simulink model "TriTiltPro_V3"  (R2019a)
settings: Solver=ode15s  StartTime=0.0  StopTime=1  RelTol=1e-3  EnableMultiTasking=on
undefined symbols (not defined in the file or in its folder): magnitude, sigbuilder_block, X, Y, Z
libraries: sm_lib x405, nesl_utility x28, simulink x13, fl_lib x7, fl_ps_legacy_lib x6, sharedtransform x1, Multibody_Multiphysics_Lib x1
(part 3 of 9)

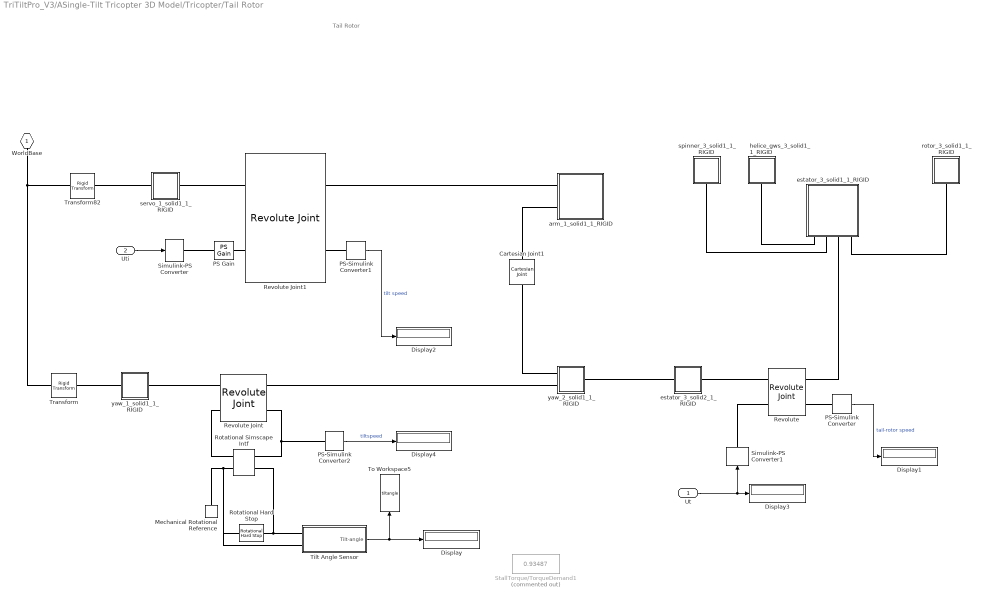
== system TriTiltPro_V3/ASingle-Tilt Tricopter 3D Model/Tricopter/Tail Rotor ==
  note: Tail Rotor
  Ut : Inport
  Uti : Inport  Port=2
  Cartesian Joint1 : sm_lib/Joints/Cartesian Joint  SenseConstraintForce=off  SenseConstraintForceX=off  SenseConstraintForceY=off  SenseConstraintForceZ=off  SenseConstraintTorque=off  SenseConstraintTorqueX=off  SenseConstraintTorqueY=off  SenseConstraintTorqueZ=off  SenseTotalForce=off  SenseTotalForceX=off  SenseTotalForceY=off  SenseTotalForceZ=off  SenseTotalTorque=off  SenseTotalTorqueX=off  SenseTotalTorqueY=off  SenseTotalTorqueZ=off  CompositeWrenchDir=FollowerOnBase  CompositeWrenchFrame=BaseFrame  PxEquilibriumPosition=0  PxEquilibriumPositionUnits=m  PxSpringStiffness=0  PxSpringStiffnessUnits=N/m  PxDampingCoefficient=0  PxDampingCoefficientUnits=N/(m/s)  PxTorqueActuationMode=NoTorque  PxMotionActuationMode=ComputedMotion  PxSensePosition=off  PxSenseVelocity=off  PxSenseAcceleration=off  PxSenseTorqueForce=off  PxSenseLowerLimitTorqueForce=off  PxSenseUpperLimitTorqueForce=off  PxLowerLimitSpecify=off  PxLowerLimitBound=-1  PxLowerLimitBoundUnits=m  PxLowerLimitStiffness=1e6  PxLowerLimitStiffnessUnits=N/m  PxLowerLimitDamping=1e3  PxLowerLimitDampingUnits=N/(m/s)  PxLowerLimitTransitionRegionWidth=1e-4  PxLowerLimitTransitionRegionWidthUnits=m  PxUpperLimitSpecify=off  PxUpperLimitBound=1  PxUpperLimitBoundUnits=m  PxUpperLimitStiffness=1e6  PxUpperLimitStiffnessUnits=N/m  PxUpperLimitDamping=1e3  PxUpperLimitDampingUnits=N/(m/s)  PxUpperLimitTransitionRegionWidth=1e-4  PxUpperLimitTransitionRegionWidthUnits=m  PxPositionTargetSpecify=off  PxPositionTargetPriority=Low  PxPositionTargetValue=-0.0011181976595044071  PxPositionTargetValueUnits=m  PxVelocityTargetSpecify=off  PxVelocityTargetPriority=High  PxVelocityTargetValue=0  PxVelocityTargetValueUnits=m/s  PyEquilibriumPosition=0  PyEquilibriumPositionUnits=m  PySpringStiffness=0  PySpringStiffnessUnits=N/m  PyDampingCoefficient=0  PyDampingCoefficientUnits=N/(m/s)  PyTorqueActuationMode=NoTorque  PyMotionActuationMode=ComputedMotion  PySensePosition=off  PySenseVelocity=off  PySenseAcceleration=off  PySenseTorqueForce=off  PySenseLowerLimitTorqueForce=off  PySenseUpperLimitTorqueForce=off  PyLowerLimitSpecify=off  PyLowerLimitBound=-1  PyLowerLimitBoundUnits=m  PyLowerLimitStiffness=1e6  PyLowerLimitStiffnessUnits=N/m  PyLowerLimitDamping=1e3  PyLowerLimitDampingUnits=N/(m/s)  PyLowerLimitTransitionRegionWidth=1e-4  PyLowerLimitTransitionRegionWidthUnits=m  PyUpperLimitSpecify=off  PyUpperLimitBound=1  PyUpperLimitBoundUnits=m  PyUpperLimitStiffness=1e6  PyUpperLimitStiffnessUnits=N/m  PyUpperLimitDamping=1e3  PyUpperLimitDampingUnits=N/(m/s)  PyUpperLimitTransitionRegionWidth=1e-4  PyUpperLimitTransitionRegionWidthUnits=m  PyPositionTargetSpecify=off  PyPositionTargetPriority=Low  PyPositionTargetValue=7.2724548069575946e-05  PyPositionTargetValueUnits=m  PyVelocityTargetSpecify=off  PyVelocityTargetPriority=High  PyVelocityTargetValue=0  PyVelocityTargetValueUnits=m/s  PzEquilibriumPosition=0  PzEquilibriumPositionUnits=m  PzSpringStiffness=0  PzSpringStiffnessUnits=N/m  PzDampingCoefficient=0  PzDampingCoefficientUnits=N/(m/s)  PzTorqueActuationMode=NoTorque  PzMotionActuationMode=ComputedMotion  PzSensePosition=off  PzSenseVelocity=off  PzSenseAcceleration=off  PzSenseTorqueForce=off  PzSenseLowerLimitTorqueForce=off  PzSenseUpperLimitTorqueForce=off  PzLowerLimitSpecify=off  PzLowerLimitBound=-1  PzLowerLimitBoundUnits=m  PzLowerLimitStiffness=1e6  PzLowerLimitStiffnessUnits=N/m  PzLowerLimitDamping=1e3  PzLowerLimitDampingUnits=N/(m/s)  PzLowerLimitTransitionRegionWidth=1e-4  PzLowerLimitTransitionRegionWidthUnits=m  PzUpperLimitSpecify=off  PzUpperLimitBound=1  PzUpperLimitBoundUnits=m  PzUpperLimitStiffness=1e6  PzUpperLimitStiffnessUnits=N/m  PzUpperLimitDamping=1e3  PzUpperLimitDampingUnits=N/(m/s)  PzUpperLimitTransitionRegionWidth=1e-4  PzUpperLimitTransitionRegionWidthUnits=m  PzPositionTargetSpecify=on  PzPositionTargetPriority=High  PzPositionTargetValue=-3.6271878084718665e-16  PzPositionTargetValueUnits=m  PzVelocityTargetSpecify=off  PzVelocityTargetPriority=High  PzVelocityTargetValue=0  PzVelocityTargetValueUnits=m/s
  Display{,1..4} (5 alike) : Display
  Mechanical Rotational Reference : fl_lib/Mechanical/Rotational Elements/Mechanical Rotational Reference
  PS Gain : fl_lib/Physical Signals/Functions/PS Gain  gain=1
  PS-Simulink Converter : nesl_utility/PS-Simulink Converter  PhysicalDomain=network_engine_domain  SubClassName=ps_output  LeftPortType=input  RightPortType=output  PseudoPeriodic=off  Frequencies=[]  Unit=rpm  AffineConversion=off
  PS-Simulink Converter1 : nesl_utility/PS-Simulink Converter  PhysicalDomain=network_engine_domain  SubClassName=ps_output  LeftPortType=input  RightPortType=output  PseudoPeriodic=off  Frequencies=[]  Unit=rpm  AffineConversion=off
  PS-Simulink Converter2 : nesl_utility/PS-Simulink Converter  PhysicalDomain=network_engine_domain  SubClassName=ps_output  LeftPortType=input  RightPortType=output  PseudoPeriodic=off  Frequencies=[]  Unit=rpm  AffineConversion=off
  Revolute : sm_lib/Joints/Revolute Joint  SenseConstraintForce=off  SenseConstraintForceX=off  SenseConstraintForceY=off  SenseConstraintForceZ=off  SenseConstraintTorque=off  SenseConstraintTorqueX=off  SenseConstraintTorqueY=off  SenseConstraintTorqueZ=off  SenseTotalForce=off  SenseTotalForceX=off  SenseTotalForceY=off  SenseTotalForceZ=off  SenseTotalTorque=off  SenseTotalTorqueX=off  SenseTotalTorqueY=off  SenseTotalTorqueZ=off  CompositeWrenchDir=FollowerOnBase  CompositeWrenchFrame=BaseFrame  EquilibriumPosition=0  EquilibriumPositionUnits=rad  SpringStiffness=0  SpringStiffnessUnits=m*N/rad  DampingCoefficient=0  DampingCoefficientUnits=m*s*N/rad  TorqueActuationMode=InputTorque  MotionActuationMode=ComputedMotion  SensePosition=off  SenseVelocity=on  SenseAcceleration=off  SenseTorqueForce=off  SenseLowerLimitTorqueForce=off  SenseUpperLimitTorqueForce=off  LowerLimitSpecify=off  LowerLimitBound=-90  LowerLimitBoundUnits=deg  LowerLimitStiffness=1e4  LowerLimitStiffnessUnits=N*m/deg  LowerLimitDamping=10  LowerLimitDampingUnits=N*m/(deg/s)  LowerLimitTransitionRegionWidth=0.1  LowerLimitTransitionRegionWidthUnits=deg  UpperLimitSpecify=off  UpperLimitBound=90  UpperLimitBoundUnits=deg  UpperLimitStiffness=1e4  UpperLimitStiffnessUnits=N*m/deg  UpperLimitDamping=10  UpperLimitDampingUnits=N*m/(deg/s)  UpperLimitTransitionRegionWidth=0.1  UpperLimitTransitionRegionWidthUnits=deg  PositionTargetSpecify=on  PositionTargetPriority=Low  PositionTargetValue=57.946376852281944  PositionTargetValueUnits=deg  VelocityTargetSpecify=off  VelocityTargetPriority=High  VelocityTargetValue=0  VelocityTargetValueUnits=deg/s
  Revolute Joint : sm_lib/Joints/Revolute Joint  SenseConstraintForce=off  SenseConstraintForceX=off  SenseConstraintForceY=off  SenseConstraintForceZ=off  SenseConstraintTorque=off  SenseConstraintTorqueX=off  SenseConstraintTorqueY=off  SenseConstraintTorqueZ=off  SenseTotalForce=off  SenseTotalForceX=off  SenseTotalForceY=off  SenseTotalForceZ=off  SenseTotalTorque=off  SenseTotalTorqueX=off  SenseTotalTorqueY=off  SenseTotalTorqueZ=off  CompositeWrenchDir=FollowerOnBase  CompositeWrenchFrame=BaseFrame  EquilibriumPosition=0  EquilibriumPositionUnits=deg  SpringStiffness=0  SpringStiffnessUnits=N*m/deg  DampingCoefficient=0  DampingCoefficientUnits=N*m/(deg/s)  TorqueActuationMode=InputTorque  MotionActuationMode=ComputedMotion  SensePosition=off  SenseVelocity=on  SenseAcceleration=off  SenseTorqueForce=off  SenseLowerLimitTorqueForce=off  SenseUpperLimitTorqueForce=off  LowerLimitSpecify=off  LowerLimitBound=-90  LowerLimitBoundUnits=deg  LowerLimitStiffness=1e4  LowerLimitStiffnessUnits=N*m/deg  LowerLimitDamping=10  LowerLimitDampingUnits=N*m/(deg/s)  LowerLimitTransitionRegionWidth=0.1  LowerLimitTransitionRegionWidthUnits=deg  UpperLimitSpecify=off  UpperLimitBound=90  UpperLimitBoundUnits=deg  UpperLimitStiffness=1e4  UpperLimitStiffnessUnits=N*m/deg  UpperLimitDamping=10  UpperLimitDampingUnits=N*m/(deg/s)  UpperLimitTransitionRegionWidth=0.1  UpperLimitTransitionRegionWidthUnits=deg  PositionTargetSpecify=off  PositionTargetPriority=Low  PositionTargetValue=0  PositionTargetValueUnits=deg  VelocityTargetSpecify=off  VelocityTargetPriority=High  VelocityTargetValue=0  VelocityTargetValueUnits=deg/s
  Revolute Joint1 : sm_lib/Joints/Revolute Joint  SenseConstraintForce=off  SenseConstraintForceX=off  SenseConstraintForceY=off  SenseConstraintForceZ=off  SenseConstraintTorque=off  SenseConstraintTorqueX=off  SenseConstraintTorqueY=off  SenseConstraintTorqueZ=off  SenseTotalForce=off  SenseTotalForceX=off  SenseTotalForceY=off  SenseTotalForceZ=off  SenseTotalTorque=off  SenseTotalTorqueX=off  SenseTotalTorqueY=off  SenseTotalTorqueZ=off  CompositeWrenchDir=FollowerOnBase  CompositeWrenchFrame=BaseFrame  EquilibriumPosition=0  EquilibriumPositionUnits=deg  SpringStiffness=0  SpringStiffnessUnits=N*m/deg  DampingCoefficient=0  DampingCoefficientUnits=N*m/(deg/s)  TorqueActuationMode=InputTorque  MotionActuationMode=ComputedMotion  SensePosition=off  SenseVelocity=on  SenseAcceleration=off  SenseTorqueForce=off  SenseLowerLimitTorqueForce=off  SenseUpperLimitTorqueForce=off  LowerLimitSpecify=off  LowerLimitBound=-90  LowerLimitBoundUnits=deg  LowerLimitStiffness=1e4  LowerLimitStiffnessUnits=N*m/deg  LowerLimitDamping=10  LowerLimitDampingUnits=N*m/(deg/s)  LowerLimitTransitionRegionWidth=0.1  LowerLimitTransitionRegionWidthUnits=deg  UpperLimitSpecify=off  UpperLimitBound=90  UpperLimitBoundUnits=deg  UpperLimitStiffness=1e4  UpperLimitStiffnessUnits=N*m/deg  UpperLimitDamping=10  UpperLimitDampingUnits=N*m/(deg/s)  UpperLimitTransitionRegionWidth=0.1  UpperLimitTransitionRegionWidthUnits=deg  PositionTargetSpecify=on  PositionTargetPriority=Low  PositionTargetValue=7.4422433437709268  PositionTargetValueUnits=deg  VelocityTargetSpecify=off  VelocityTargetPriority=High  VelocityTargetValue=0  VelocityTargetValueUnits=deg/s
  Rotational Simscape Intf : Multibody_Multiphysics_Lib/Interfaces/Rotational Simscape Intf  SystemSampleTime=-1
      settings: SourceProductName=Simscape Multibody Multiphysics Library
  Rotational Hard Stop : fl_lib/Mechanical/Rotational Elements/Rotational Hard Stop  upper_bnd=225 deg  lower_bnd=135 deg  stiff_up=2e6 N*m/rad  stiff_low=2e6 N*m/rad  D_up=0.000001 N*m/(rad/s)  D_low=0.000001 N*m/(rad/s)  model=3  transition=0.001 rad  w_specify=off  w_priority=High  w=0 rad/s  w_nominal_specify=off  w_nominal_unit=rad/s  w_nominal_value=1  t_specify=off  t_priority=High  t=0 N*m  t_nominal_specify=off  t_nominal_unit=N*m  t_nominal_value=1  phi_specify=on  phi_priority=High  phi=180 deg  phi_nominal_specify=off  phi_nominal_unit=rad  phi_nominal_value=1
      settings: SourceProductName=Simscape  SourceProductBaseCode=SS
  Simulink-PS Converter : nesl_utility/Simulink-PS Converter  PhysicalDomain=network_engine_domain  SubClassName=ps_input  LeftPortType=input  RightPortType=output  PseudoPeriodic=off  Frequencies=[]  NoiseDistribution=none  NoiseParameters=[]  Unit=N*m  AffineConversion=off  FilteringAndDerivatives=zero  SimscapeFilterOrder=1  InputFilterTimeConstant=0.001  UdotUserProvided=1
  Simulink-PS Converter1 : nesl_utility/Simulink-PS Converter  PhysicalDomain=network_engine_domain  SubClassName=ps_input  LeftPortType=input  RightPortType=output  PseudoPeriodic=off  Frequencies=[]  NoiseDistribution=none  NoiseParameters=[]  Unit=N*m  AffineConversion=off  FilteringAndDerivatives=zero  SimscapeFilterOrder=1  InputFilterTimeConstant=0.001  UdotUserProvided=1
  StallTorque/TorqueDemand1 : Constant  Commented=on  Value=0.93487
  Tilt Angle Sensor : Subsystem
  To Workspace5 : ToWorkspace  VariableName=tiltangle  SampleTime=-1
  Transform : sm_lib/Frames and Transforms/Rigid Transform  TranslationMethod=None  TranslationStandardOffset=0  TranslationLengthUnit=m  TranslationStandardAxis=+Z  TranslationCartesianOffset=[0 0 0]  TranslationROffset=0  TranslationROffsetUnits=m  TranslationZOffset=0  TranslationZOffsetUnits=m  TranslationThetaOffset=0  TranslationThetaOffsetUnits=deg  RotationMethod=None  RotationAngleUnits=deg  RotationStandardAxis=+Z  RotationAngle=0.0  RotationArbitraryAxis=[0 0 1]  FollAlignAxisA=+X  BaseAlignAxisA=+Y  FollAlignAxisB=+Y  BaseAlignAxisB=+Z  RotationSequenceAxes=FollowerAxes  RotationSequence=XYX  RotationSequenceAngles=[0 0 0]  RotationSequenceAnglesUnits=deg  RotationMatrix=[1 0 0; 0 1 0; 0 0 1]
  Transform82 : sm_lib/Frames and Transforms/Rigid Transform  TranslationMethod=None  TranslationStandardOffset=0  TranslationLengthUnit=m  TranslationStandardAxis=+Z  TranslationCartesianOffset=[0 0 0]  TranslationROffset=0  TranslationROffsetUnits=m  TranslationZOffset=0  TranslationZOffsetUnits=m  TranslationThetaOffset=0  TranslationThetaOffsetUnits=deg  RotationMethod=None  RotationAngleUnits=deg  RotationStandardAxis=+Z  RotationAngle=0.0  RotationArbitraryAxis=[0 0 1]  FollAlignAxisA=+X  BaseAlignAxisA=+Y  FollAlignAxisB=+Y  BaseAlignAxisB=+Z  RotationSequenceAxes=FollowerAxes  RotationSequence=XYX  RotationSequenceAngles=[0 0 0]  RotationSequenceAnglesUnits=deg  RotationMatrix=[1 0 0; 0 1 0; 0 0 1]
  arm_1_solid1_1_RIGID : Subsystem
  estator_3_solid1_1_RIGID : Subsystem
  estator_3_solid2_1_RIGID : Subsystem
  helice_gws_3_solid1_1_RIGID : Subsystem
  rotor_3_solid1_1_RIGID : Subsystem
  servo_1_solid1_1_RIGID : Subsystem
  spinner_3_solid1_1_RIGID : Subsystem
  yaw_1_solid1_1_RIGID : Subsystem
  yaw_2_solid1_1_RIGID : Subsystem
  WorldBase : PMIOPort  Side=Right
  wires:
  Tilt Angle Sensor/1(Tilt-angle) -> To Workspace5/1, Display/1
  PS-Simulink Converter/1 -> Display1/1  "tail-rotor speed"
  Uti/1 -> Simulink-PS Converter/1
  Ut/1 -> Display3/1, Simulink-PS Converter1/1
  PS-Simulink Converter1/1 -> Display2/1  "tilt speed"
  PS-Simulink Converter2/1 -> Display4/1  "tiltspeed"
  connections:
  Transform/RConn1 -- yaw_1_solid1_1_RIGID/LConn1
  estator_3_solid2_1_RIGID/LConn1 -- yaw_2_solid1_1_RIGID/RConn1
  Transform82/RConn1 -- servo_1_solid1_1_RIGID/LConn1
  WorldBase/RConn1 -- Transform82/LConn1 -- Transform/LConn1
  Revolute Joint/LConn1 -- yaw_1_solid1_1_RIGID/RConn1
  Revolute Joint/RConn1 -- yaw_2_solid1_1_RIGID/LConn2
  Revolute Joint1/LConn1 -- servo_1_solid1_1_RIGID/RConn1
  Revolute Joint1/RConn1 -- arm_1_solid1_1_RIGID/LConn1
  Tilt Angle Sensor/LConn2 -- Rotational Hard Stop/RConn1 -- Rotational Simscape Intf/LConn2 -- Mechanical Rotational Reference/LConn1
  estator_3_solid2_1_RIGID/RConn1 -- Revolute/LConn1
  PS-Simulink Converter/LConn1 -- Revolute/RConn2
  PS Gain/RConn1 -- Revolute Joint1/LConn2
  Simulink-PS Converter/RConn1 -- PS Gain/LConn1
  arm_1_solid1_1_RIGID/LConn2 -- Cartesian Joint1/LConn1
  Tilt Angle Sensor/LConn1 -- Rotational Simscape Intf/RConn2 -- Rotational Hard Stop/LConn1
  Revolute Joint/RConn2 -- Rotational Simscape Intf/RConn1 -- PS-Simulink Converter2/LConn1
  Rotational Simscape Intf/LConn1 -- Revolute Joint/LConn2
  Simulink-PS Converter1/RConn1 -- Revolute/LConn2
  PS-Simulink Converter1/LConn1 -- Revolute Joint1/RConn2
  Cartesian Joint1/RConn1 -- yaw_2_solid1_1_RIGID/LConn1
  helice_gws_3_solid1_1_RIGID/LConn1 -- estator_3_solid1_1_RIGID/LConn1
  spinner_3_solid1_1_RIGID/LConn1 -- estator_3_solid1_1_RIGID/LConn2
  rotor_3_solid1_1_RIGID/LConn1 -- estator_3_solid1_1_RIGID/LConn4
  estator_3_solid1_1_RIGID/LConn3 -- Revolute/RConn1

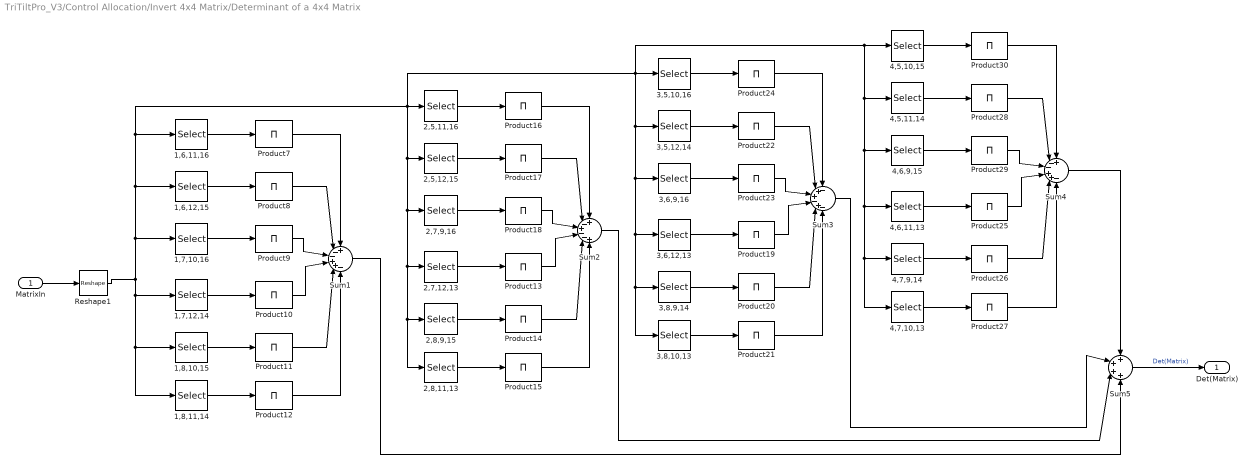
== system TriTiltPro_V3/Control Allocation/Invert 4x4 Matrix/Determinant of a 4x4 Matrix ==
  MatrixIn : Inport
  1,6,11,16 : Selector  InputPortWidth=16  IndexOptions=Index vector (dialog)  Indices=[1 6 11 16]  OutputSizes=1
  1,6,12,15 : Selector  InputPortWidth=16  IndexOptions=Index vector (dialog)  Indices=[1 6 12 15]  OutputSizes=1
  1,7,10,16 : Selector  InputPortWidth=16  IndexOptions=Index vector (dialog)  Indices=[1 7 10 16]  OutputSizes=1
  1,7,12,14 : Selector  InputPortWidth=16  IndexOptions=Index vector (dialog)  Indices=[1 7 10 16]  OutputSizes=1
  1,8,10,15 : Selector  InputPortWidth=16  IndexOptions=Index vector (dialog)  Indices=[1 7 10 16]  OutputSizes=1
  1,8,11,14 : Selector  InputPortWidth=16  IndexOptions=Index vector (dialog)  Indices=[1 7 10 16]  OutputSizes=1
  2,5,11,16 : Selector  InputPortWidth=16  IndexOptions=Index vector (dialog)  Indices=[2 5 11 16]  OutputSizes=1
  2,5,12,15 : Selector  InputPortWidth=16  IndexOptions=Index vector (dialog)  Indices=[2 5 12 15]  OutputSizes=1
  2,7,12,13 : Selector  InputPortWidth=16  IndexOptions=Index vector (dialog)  Indices=[2 7 12 13]  OutputSizes=1
  2,7,9,16 : Selector  InputPortWidth=16  IndexOptions=Index vector (dialog)  Indices=[2 7 9 16]  OutputSizes=1
  2,8,11,13 : Selector  InputPortWidth=16  IndexOptions=Index vector (dialog)  Indices=[2 8 11 13]  OutputSizes=1
  2,8,9,15 : Selector  InputPortWidth=16  IndexOptions=Index vector (dialog)  Indices=[2 8 9 15]  OutputSizes=1
  3,5,10,16 : Selector  InputPortWidth=16  IndexOptions=Index vector (dialog)  Indices=[3 5 10 16]  OutputSizes=1
  3,5,12,14 : Selector  InputPortWidth=16  IndexOptions=Index vector (dialog)  Indices=[3 5 12 14]  OutputSizes=1
  3,6,12,13 : Selector  InputPortWidth=16  IndexOptions=Index vector (dialog)  Indices=[3 6 12 13]  OutputSizes=1
  3,6,9,16 : Selector  InputPortWidth=16  IndexOptions=Index vector (dialog)  Indices=[3 6 9 16]  OutputSizes=1
  3,8,10,13 : Selector  InputPortWidth=16  IndexOptions=Index vector (dialog)  Indices=[3 8 10 13]  OutputSizes=1
  3,8,9,14 : Selector  InputPortWidth=16  IndexOptions=Index vector (dialog)  Indices=[3 8 9 14]  OutputSizes=1
  4,5,10,15 : Selector  InputPortWidth=16  IndexOptions=Index vector (dialog)  Indices=[4 5 10 15]  OutputSizes=1
  4,5,11,14 : Selector  InputPortWidth=16  IndexOptions=Index vector (dialog)  Indices=[4 5 11 14]  OutputSizes=1
  4,6,11,13 : Selector  InputPortWidth=16  IndexOptions=Index vector (dialog)  Indices=[4 6 11 13]  OutputSizes=1
  4,6,9,15 : Selector  InputPortWidth=16  IndexOptions=Index vector (dialog)  Indices=[4 6 9 15]  OutputSizes=1
  4,7,10,13 : Selector  InputPortWidth=16  IndexOptions=Index vector (dialog)  Indices=[4 7 10 13]  OutputSizes=1
  4,7,9,14 : Selector  InputPortWidth=16  IndexOptions=Index vector (dialog)  Indices=[4 7 9 14]  OutputSizes=1
  Product{7..30} (24 alike) : Product  Inputs=1  SaturateOnIntegerOverflow=on  OutDataTypeStr=Inherit: Same as first input
  Reshape1 : Reshape  OutputDimensionality=Row vector (2-D)  OutputDimensions=[4,4]
  Sum1 : Sum  Inputs=+--++-  SaturateOnIntegerOverflow=on
  Sum2 : Sum  Inputs=+-+--+  SaturateOnIntegerOverflow=on
  Sum3 : Sum  Inputs=-++-+-  SaturateOnIntegerOverflow=on
  Sum4 : Sum  Inputs=+--++-  SaturateOnIntegerOverflow=on
  Sum5 : Sum  Inputs=++++  SaturateOnIntegerOverflow=on
  Det(Matrix) : Outport
  wires:
  Product8/1 -> Sum1/2
  1,6,11,16/1 -> Product7/1
  3,5,10,16/1 -> Product24/1
  Reshape1/1 -> 1,6,12,15/1, 3,5,12,14/1, 3,8,10,13/1, 3,8,9,14/1, 3,6,12,13/1, 3,6,9,16/1, 4,6,9,15/1, 4,7,10,13/1, 4,7,9,14/1, 4,6,11,13/1, 4,5,11,14/1, 4,5,10,15/1, 3,5,10,16/1, 2,7,9,16/1, 2,8,11,13/1, 2,8,9,15/1, 2,7,12,13/1, 2,5,12,15/1, 2,5,11,16/1, 1,6,11,16/1, 1,7,10,16/1, 1,7,12,14/1, 1,8,11,14/1, 1,8,10,15/1
  1,8,10,15/1 -> Product11/1
  Product10/1 -> Sum1/4
  1,7,10,16/1 -> Product9/1
  Product28/1 -> Sum4/2
  Product25/1 -> Sum4/4
  4,7,10,13/1 -> Product27/1
  Product26/1 -> Sum4/5
  4,6,11,13/1 -> Product25/1
  Product29/1 -> Sum4/3
  4,7,9,14/1 -> Product26/1
  4,6,9,15/1 -> Product29/1
  Product30/1 -> Sum4/1
  4,5,10,15/1 -> Product30/1
  4,5,11,14/1 -> Product28/1
  Product27/1 -> Sum4/6
  2,8,9,15/1 -> Product14/1
  Product13/1 -> Sum2/4
  Product14/1 -> Sum2/5
  1,7,12,14/1 -> Product10/1
  Product17/1 -> Sum2/2
  2,7,12,13/1 -> Product13/1
  Product18/1 -> Sum2/3
  Product15/1 -> Sum2/6
  2,7,9,16/1 -> Product18/1
  2,5,11,16/1 -> Product16/1
  Product16/1 -> Sum2/1
  2,5,12,15/1 -> Product17/1
  2,8,11,13/1 -> Product15/1
  Sum4/1 -> Sum5/1
  1,6,12,15/1 -> Product8/1
  Product11/1 -> Sum1/5
  Sum5/1 -> Det(Matrix)/1  "Det(Matrix)"
  Sum3/1 -> Sum5/2
  Sum2/1 -> Sum5/3
  Product24/1 -> Sum3/1
  Sum1/1 -> Sum5/4
  Product9/1 -> Sum1/3
  Product7/1 -> Sum1/1
  Product23/1 -> Sum3/3
  3,8,9,14/1 -> Product20/1
  Product22/1 -> Sum3/2
  Product19/1 -> Sum3/4
  3,8,10,13/1 -> Product21/1
  Product20/1 -> Sum3/5
  Product21/1 -> Sum3/6
  3,6,12,13/1 -> Product19/1
  3,5,12,14/1 -> Product22/1
  3,6,9,16/1 -> Product23/1
  1,8,11,14/1 -> Product12/1
  Product12/1 -> Sum1/6
  MatrixIn/1 -> Reshape1/1

== system TriTiltPro_V3/Reference Inputs/Inputs1/Signal Builder ==
  Demux : Demux  Tag=STV Demux
  FromWs : FromWorkspace  Tag=STV FromWs  VariableName=tuvar  SampleTime=0
      SigBuilderData=|
      | common.afterFinalStr = 'Extrapolate'
      | common.sampleTime = '0'
      | dataSet.timeRange = [0 2]
      | dataSet.name = 'Group 1'
      | sbobj.Groups.Name = 'Group 1'
      | sbobj.Groups.Signals(1).Name = 'Test Altitude'
      | sbobj.Groups.Signals(1).XData = [0 0.2 0.4 0.6 0.8 2]
      | sbobj.Groups.Signals(1).YData = [0 0 0 0 0 0]
      | sbobj.Groups.Signals(2).Name = 'Test Roll'
      | sbobj.Groups.Signals(2).XData = [0 0.995 2]
      | sbobj.Groups.Signals(2).YData = [0 0 0]
      | sbobj.Groups.Signals(3).Name = 'Test Pitch'
      | sbobj.Groups.Signals(3).XData = [0 2]
      | sbobj.Groups.Signals(3).YData = [0 0]
      | sbobj.Groups.Signals(4).Name = 'Test Yaw'
      | sbobj.Groups.Signals(4).XData = [0 2]
      | sbobj.Groups.Signals(4).YData = [0 0]
      | sbobj.Groups.TimeRange = [0 2]
  Test Altitude : Outport  Tag=STV Outport
  Test Roll : Outport  Tag=STV Outport  Port=2
  Test Pitch : Outport  Tag=STV Outport  Port=3
  Test Yaw : Outport  Tag=STV Outport  Port=4
  wires:
  FromWs/1 -> Demux/1
  Demux/1 -> Test Altitude/1
  Demux/2 -> Test Roll/1
  Demux/3 -> Test Pitch/1
  Demux/4 -> Test Yaw/1

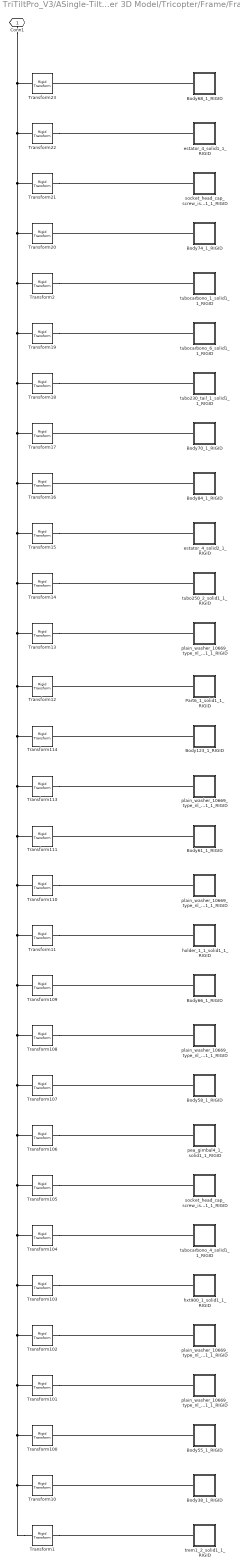
== system TriTiltPro_V3/ASingle-Tilt Tricopter 3D Model/Tricopter/Frame/Frame B ==
  Body123_1_RIGID : Subsystem
  Body38_1_RIGID : Subsystem
  Body55_1_RIGID : Subsystem
  Body58_1_RIGID : Subsystem
  Body61_1_RIGID : Subsystem
  Body66_1_RIGID : Subsystem
  Body68_1_RIGID : Subsystem
  Body70_1_RIGID : Subsystem
  Body74_1_RIGID : Subsystem
  Body84_1_RIGID : Subsystem
  Part6_1_solid1_1_RIGID : Subsystem
  Transform{1..2,10..23,100..111,113..114} (30 alike) : sm_lib/Frames and Transforms/Rigid Transform  TranslationMethod=None  TranslationStandardOffset=0  TranslationLengthUnit=m  TranslationStandardAxis=+Z  TranslationCartesianOffset=[0 0 0]  TranslationROffset=0  TranslationROffsetUnits=m  TranslationZOffset=0  TranslationZOffsetUnits=m  TranslationThetaOffset=0  TranslationThetaOffsetUnits=deg  RotationMethod=None  RotationAngleUnits=deg  RotationStandardAxis=+Z  RotationAngle=0.0  RotationArbitraryAxis=[0 0 1]  FollAlignAxisA=+X  BaseAlignAxisA=+Y  FollAlignAxisB=+Y  BaseAlignAxisB=+Z  RotationSequenceAxes=FollowerAxes  RotationSequence=XYX  RotationSequenceAngles=[0 0 0]  RotationSequenceAnglesUnits=deg  RotationMatrix=[1 0 0; 0 1 0; 0 0 1]
  estator_4_solid1_1_RIGID : Subsystem
  estator_4_solid2_1_RIGID : Subsystem
  holder_1_1_solid1_1_RIGID : Subsystem
  hxt900_1_solid1_1_RIGID : Subsystem
  pea_gimbal4_1_solid1_1_RIGID : Subsystem
  plain_washer_10669_type_nl_iso_10_solid1_1_RIGID : Subsystem
  plain_washer_10669_type_nl_iso_11_solid1_1_RIGID : Subsystem
  plain_washer_10669_type_nl_iso_12_solid1_1_RIGID : Subsystem
  plain_washer_10669_type_nl_iso_13_solid1_1_RIGID : Subsystem
  plain_washer_10669_type_nl_iso_14_solid1_1_RIGID : Subsystem
  plain_washer_10669_type_nl_iso_4_solid1_1_RIGID : Subsystem
  socket_head_cap_screw_iso_3_solid1_1_RIGID : Subsystem
  socket_head_cap_screw_iso_4_solid1_1_RIGID : Subsystem
  trem1_2_solid1_1_RIGID : Subsystem
  tubo230_tail_1_solid1_1_RIGID : Subsystem
  tubo250_2_solid1_1_RIGID : Subsystem
  tubocarbono_1_solid1_1_RIGID : Subsystem
  tubocarbono_4_solid1_1_RIGID : Subsystem
  tubocarbono_6_solid1_1_RIGID : Subsystem
  Conn1 : PMIOPort  Side=Right
  connections:
  Transform19/RConn1 -- tubocarbono_6_solid1_1_RIGID/LConn1
  Transform21/RConn1 -- socket_head_cap_screw_iso_3_solid1_1_RIGID/LConn1
  Body74_1_RIGID/LConn1 -- Transform20/RConn1
  Transform22/RConn1 -- estator_4_solid1_1_RIGID/LConn1
  Body68_1_RIGID/LConn1 -- Transform23/RConn1
  Part6_1_solid1_1_RIGID/LConn1 -- Transform12/RConn1
  Transform13/RConn1 -- plain_washer_10669_type_nl_iso_10_solid1_1_RIGID/LConn1
  Transform14/RConn1 -- tubo250_2_solid1_1_RIGID/LConn1
  Transform11/RConn1 -- holder_1_1_solid1_1_RIGID/LConn1
  Transform15/RConn1 -- estator_4_solid2_1_RIGID/LConn1
  Body84_1_RIGID/LConn1 -- Transform16/RConn1
  Body38_1_RIGID/LConn1 -- Transform10/RConn1
  Body70_1_RIGID/LConn1 -- Transform17/RConn1
  Transform18/RConn1 -- tubo230_tail_1_solid1_1_RIGID/LConn1
  Transform1/RConn1 -- trem1_2_solid1_1_RIGID/LConn1
  Transform2/RConn1 -- tubocarbono_1_solid1_1_RIGID/LConn1
  Transform103/RConn1 -- hxt900_1_solid1_1_RIGID/LConn1
  Transform110/RConn1 -- plain_washer_10669_type_nl_iso_11_solid1_1_RIGID/LConn1
  Body58_1_RIGID/LConn1 -- Transform107/RConn1
  Transform105/RConn1 -- socket_head_cap_screw_iso_4_solid1_1_RIGID/LConn1
  Transform113/RConn1 -- plain_washer_10669_type_nl_iso_4_solid1_1_RIGID/LConn1
  Body123_1_RIGID/LConn1 -- Transform114/RConn1
  Transform102/RConn1 -- plain_washer_10669_type_nl_iso_13_solid1_1_RIGID/LConn1
  Body55_1_RIGID/LConn1 -- Transform100/RConn1
  Transform101/RConn1 -- plain_washer_10669_type_nl_iso_14_solid1_1_RIGID/LConn1
  Body66_1_RIGID/LConn1 -- Transform109/RConn1
  Transform106/RConn1 -- pea_gimbal4_1_solid1_1_RIGID/LConn1
  Body61_1_RIGID/LConn1 -- Transform111/RConn1
  Transform104/RConn1 -- tubocarbono_4_solid1_1_RIGID/LConn1
  Transform108/RConn1 -- plain_washer_10669_type_nl_iso_12_solid1_1_RIGID/LConn1
  Transform1/LConn1 -- Transform10/LConn1 -- Transform100/LConn1 -- Transform101/LConn1 -- Transform102/LConn1 -- Transform103/LConn1 -- Transform104/LConn1 -- Transform105/LConn1 -- Transform106/LConn1 -- Transform107/LConn1 -- Transform108/LConn1 -- Transform109/LConn1 -- Transform11/LConn1 -- Transform110/LConn1 -- Transform111/LConn1 -- Transform113/LConn1 -- Transform114/LConn1 -- Transform12/LConn1 -- Transform13/LConn1 -- Transform14/LConn1 -- Transform15/LConn1 -- Transform16/LConn1 -- Transform17/LConn1 -- Transform18/LConn1 -- Transform19/LConn1 -- Transform2/LConn1 -- Transform20/LConn1 -- Transform21/LConn1 -- Transform22/LConn1 -- Transform23/LConn1 -- Conn1/RConn1

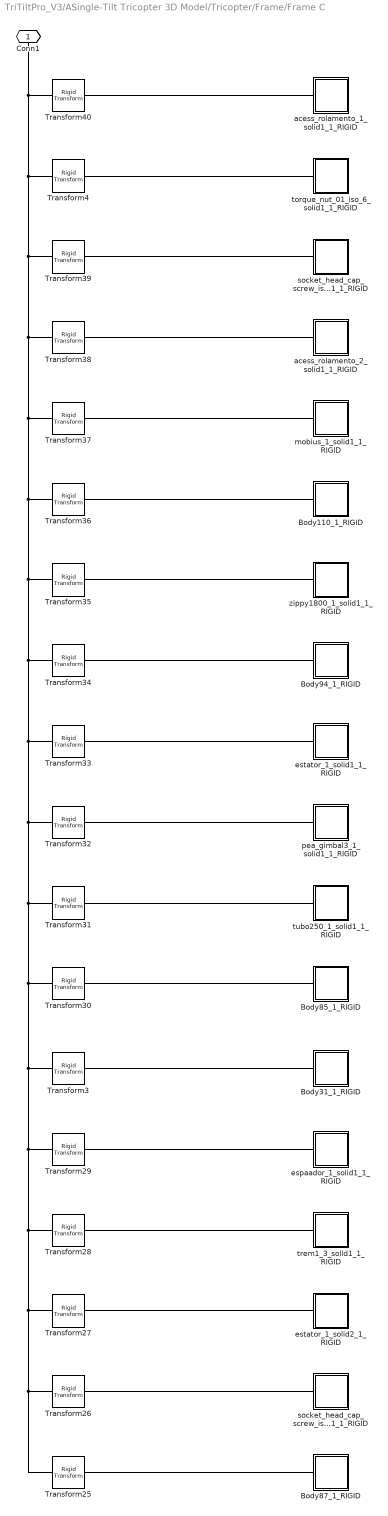
== system TriTiltPro_V3/ASingle-Tilt Tricopter 3D Model/Tricopter/Frame/Frame C ==
  Body110_1_RIGID : Subsystem
  Body31_1_RIGID : Subsystem
  Body85_1_RIGID : Subsystem
  Body87_1_RIGID : Subsystem
  Body94_1_RIGID : Subsystem
  Transform{3..4,25..40} (18 alike) : sm_lib/Frames and Transforms/Rigid Transform  TranslationMethod=None  TranslationStandardOffset=0  TranslationLengthUnit=m  TranslationStandardAxis=+Z  TranslationCartesianOffset=[0 0 0]  TranslationROffset=0  TranslationROffsetUnits=m  TranslationZOffset=0  TranslationZOffsetUnits=m  TranslationThetaOffset=0  TranslationThetaOffsetUnits=deg  RotationMethod=None  RotationAngleUnits=deg  RotationStandardAxis=+Z  RotationAngle=0.0  RotationArbitraryAxis=[0 0 1]  FollAlignAxisA=+X  BaseAlignAxisA=+Y  FollAlignAxisB=+Y  BaseAlignAxisB=+Z  RotationSequenceAxes=FollowerAxes  RotationSequence=XYX  RotationSequenceAngles=[0 0 0]  RotationSequenceAnglesUnits=deg  RotationMatrix=[1 0 0; 0 1 0; 0 0 1]
  acess_rolamento_1_solid1_1_RIGID : Subsystem
  acess_rolamento_2_solid1_1_RIGID : Subsystem
  espaador_1_solid1_1_RIGID : Subsystem
  estator_1_solid1_1_RIGID : Subsystem
  estator_1_solid2_1_RIGID : Subsystem
  mobius_1_solid1_1_RIGID : Subsystem
  pea_gimbal3_1_solid1_1_RIGID : Subsystem
  socket_head_cap_screw_iso_1_solid1_1_RIGID : Subsystem
  socket_head_cap_screw_iso_2_solid1_1_RIGID : Subsystem
  torque_nut_01_iso_6_solid1_1_RIGID : Subsystem
  trem1_3_solid1_1_RIGID : Subsystem
  tubo250_1_solid1_1_RIGID : Subsystem
  zippy1800_1_solid1_1_RIGID : Subsystem
  Conn1 : PMIOPort  Side=Right
  connections:
  Transform28/RConn1 -- trem1_3_solid1_1_RIGID/LConn1
  Transform27/RConn1 -- estator_1_solid2_1_RIGID/LConn1
  Transform29/RConn1 -- espaador_1_solid1_1_RIGID/LConn1
  Transform26/RConn1 -- socket_head_cap_screw_iso_2_solid1_1_RIGID/LConn1
  Body87_1_RIGID/LConn1 -- Transform25/RConn1
  Body85_1_RIGID/LConn1 -- Transform30/RConn1
  Transform32/RConn1 -- pea_gimbal3_1_solid1_1_RIGID/LConn1
  Transform35/RConn1 -- zippy1800_1_solid1_1_RIGID/LConn1
  Body110_1_RIGID/LConn1 -- Transform36/RConn1
  Transform31/RConn1 -- tubo250_1_solid1_1_RIGID/LConn1
  Transform33/RConn1 -- estator_1_solid1_1_RIGID/LConn1
  Body94_1_RIGID/LConn1 -- Transform34/RConn1
  Transform37/RConn1 -- mobius_1_solid1_1_RIGID/LConn1
  Transform38/RConn1 -- acess_rolamento_2_solid1_1_RIGID/LConn1
  Transform39/RConn1 -- socket_head_cap_screw_iso_1_solid1_1_RIGID/LConn1
  Transform4/RConn1 -- torque_nut_01_iso_6_solid1_1_RIGID/LConn1
  Body31_1_RIGID/LConn1 -- Transform3/RConn1
  Transform25/LConn1 -- Conn1/RConn1 -- Transform40/LConn1 -- Transform4/LConn1 -- Transform39/LConn1 -- Transform38/LConn1 -- Transform37/LConn1 -- Transform36/LConn1 -- Transform35/LConn1 -- Transform34/LConn1 -- Transform33/LConn1 -- Transform32/LConn1 -- Transform31/LConn1 -- Transform30/LConn1 -- Transform3/LConn1 -- Transform29/LConn1 -- Transform28/LConn1 -- Transform27/LConn1 -- Transform26/LConn1
  Transform40/RConn1 -- acess_rolamento_1_solid1_1_RIGID/LConn1

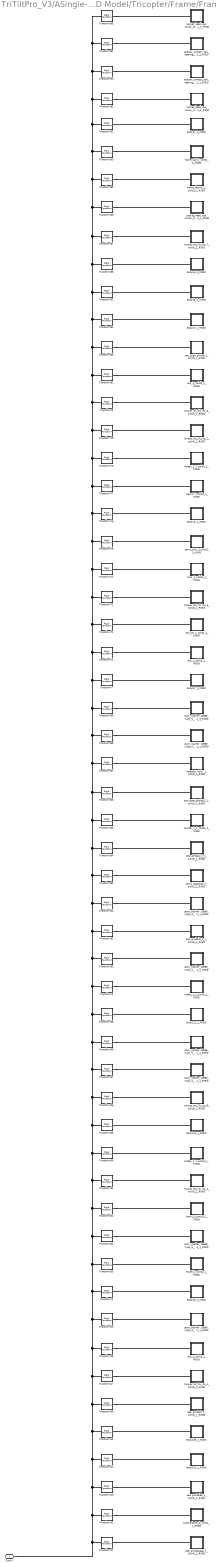
== system TriTiltPro_V3/ASingle-Tilt Tricopter 3D Model/Tricopter/Frame/Frame D ==
  Body101_1_RIGID : Subsystem
  Body106_1_RIGID : Subsystem
  Body114_1_RIGID : Subsystem
  Body121_1_RIGID : Subsystem
  Body15_1_RIGID : Subsystem
  Body19_1_RIGID : Subsystem
  Body27_1_RIGID : Subsystem
  Body29_1_RIGID : Subsystem
  Body37_1_RIGID : Subsystem
  Body44_1_RIGID : Subsystem
  Body47_1_RIGID : Subsystem
  Part6_2_solid1_1_RIGID : Subsystem
  Transform{5..8,41..69,71..79,81,83..95} (56 alike) : sm_lib/Frames and Transforms/Rigid Transform  TranslationMethod=None  TranslationStandardOffset=0  TranslationLengthUnit=m  TranslationStandardAxis=+Z  TranslationCartesianOffset=[0 0 0]  TranslationROffset=0  TranslationROffsetUnits=m  TranslationZOffset=0  TranslationZOffsetUnits=m  TranslationThetaOffset=0  TranslationThetaOffsetUnits=deg  RotationMethod=None  RotationAngleUnits=deg  RotationStandardAxis=+Z  RotationAngle=0.0  RotationArbitraryAxis=[0 0 1]  FollAlignAxisA=+X  BaseAlignAxisA=+Y  FollAlignAxisB=+Y  BaseAlignAxisB=+Z  RotationSequenceAxes=FollowerAxes  RotationSequence=XYX  RotationSequenceAngles=[0 0 0]  RotationSequenceAnglesUnits=deg  RotationMatrix=[1 0 0; 0 1 0; 0 0 1]
  angular_contact_ball_bearing_68_iso_1_solid1_1_RIGID : Subsystem
  angular_contact_ball_bearing_68_iso_3_solid1_1_RIGID : Subsystem
  camfpv_1_1_solid1_1_RIGID : Subsystem
  crius_1_solid1_1_RIGID : Subsystem
  esc_1_solid1_1_RIGID : Subsystem
  esc_2_solid1_1_RIGID : Subsystem
  esc_3_solid1_1_RIGID : Subsystem
  frame_down3_1_solid1_1_RIGID : Subsystem
  frame_up2_1_solid1_1_RIGID : Subsystem
  holder_1_2_solid1_1_RIGID : Subsystem
  holder_1_3_solid1_1_RIGID : Subsystem
  holder_1_4_solid1_1_RIGID : Subsystem
  pea_gimbal2_1_solid1_1_RIGID : Subsystem
  pea_gimbal2aaa_1_solid1_1_RIGID : Subsystem
  pea_gimbal3_2_1_solid1_1_RIGID : Subsystem
  pea_gimbal4_2_1_solid1_1_RIGID : Subsystem
  pea_gimbal55_1_solid1_1_RIGID : Subsystem
  plain_washer_10669_type_nl_iso_1_solid1_1_RIGID : Subsystem
  plain_washer_10669_type_nl_iso_2_solid1_1_RIGID : Subsystem
  plain_washer_10669_type_nl_iso_3_solid1_1_RIGID : Subsystem
  plain_washer_10669_type_nl_iso_5_solid1_1_RIGID : Subsystem
  plain_washer_10669_type_nl_iso_6_solid1_1_RIGID : Subsystem
  plain_washer_10669_type_nl_iso_7_solid1_1_RIGID : Subsystem
  plain_washer_10669_type_nl_iso_8_solid1_1_RIGID : Subsystem
  plain_washer_10669_type_nl_iso_9_solid1_1_RIGID : Subsystem
  receptor_frsky_1_solid1_1_RIGID : Subsystem
  sec_quad_gimbal2_1_solid1_1_RIGID : Subsystem
  sec_quad_gimbal_1_solid1_1_RIGID : Subsystem
  servo_arm_1_solid1_1_RIGID : Subsystem
  servo_big40x20_1_solid1_1_RIGID : Subsystem
  socket_head_cap_screw_iso_5_solid1_1_RIGID : Subsystem
  socket_head_cap_screw_iso_6_solid1_1_RIGID : Subsystem
  socket_head_cap_screw_iso_8_solid1_1_RIGID : Subsystem
  torque_nut_01_iso_1_solid1_1_RIGID : Subsystem
  torque_nut_01_iso_2_solid1_1_RIGID : Subsystem
  torque_nut_01_iso_3_solid1_1_RIGID : Subsystem
  torque_nut_01_iso_4_solid1_1_RIGID : Subsystem
  torque_nut_01_iso_5_solid1_1_RIGID : Subsystem
  torque_nut_01_iso_7_solid1_1_RIGID : Subsystem
  torque_nut_01_iso_8_solid1_1_RIGID : Subsystem
  trem1_1_solid1_1_RIGID : Subsystem
  trem1_4_solid1_1_RIGID : Subsystem
  tubocarbono_5_solid1_1_RIGID : Subsystem
  veio_30_1_solid1_1_RIGID : Subsystem
  Conn1 : PMIOPort  Side=Left
  connections:
  Transform43/RConn1 -- pea_gimbal55_1_solid1_1_RIGID/LConn1
  Transform42/RConn1 -- tubocarbono_5_solid1_1_RIGID/LConn1
  Body29_1_RIGID/LConn1 -- Transform5/RConn1
  Transform6/RConn1 -- holder_1_2_solid1_1_RIGID/LConn1
  Transform8/RConn1 -- torque_nut_01_iso_5_solid1_1_RIGID/LConn1
  Body37_1_RIGID/LConn1 -- Transform7/RConn1
  Transform81/RConn1 -- esc_2_solid1_1_RIGID/LConn1
  Transform83/RConn1 -- sec_quad_gimbal_1_solid1_1_RIGID/LConn1
  Body19_1_RIGID/LConn1 -- Transform85/RConn1
  Transform90/RConn1 -- frame_up2_1_solid1_1_RIGID/LConn1
  Transform87/RConn1 -- torque_nut_01_iso_7_solid1_1_RIGID/LConn1
  Transform88/RConn1 -- socket_head_cap_screw_iso_8_solid1_1_RIGID/LConn1
  Transform92/RConn1 -- socket_head_cap_screw_iso_5_solid1_1_RIGID/LConn1
  Body27_1_RIGID/LConn1 -- Transform84/RConn1
  Body47_1_RIGID/LConn1 -- Transform91/RConn1
  Transform93/RConn1 -- angular_contact_ball_bearing_68_iso_3_solid1_1_RIGID/LConn1
  Body44_1_RIGID/LConn1 -- Transform86/RConn1
  Transform89/RConn1 -- frame_down3_1_solid1_1_RIGID/LConn1
  Transform41/RConn1 -- pea_gimbal2aaa_1_solid1_1_RIGID/LConn1
  Transform94/RConn1 -- angular_contact_ball_bearing_68_iso_1_solid1_1_RIGID/LConn1
  Transform95/RConn1 -- socket_head_cap_screw_iso_6_solid1_1_RIGID/LConn1
  Transform62/RConn1 -- plain_washer_10669_type_nl_iso_1_solid1_1_RIGID/LConn1
  Body101_1_RIGID/LConn1 -- Transform44/RConn1
  Transform60/RConn1 -- plain_washer_10669_type_nl_iso_8_solid1_1_RIGID/LConn1
  Transform65/RConn1 -- camfpv_1_1_solid1_1_RIGID/LConn1
  Transform46/RConn1 -- pea_gimbal2_1_solid1_1_RIGID/LConn1
  Transform49/RConn1 -- plain_washer_10669_type_nl_iso_9_solid1_1_RIGID/LConn1
  Transform61/RConn1 -- pea_gimbal3_2_1_solid1_1_RIGID/LConn1
  Transform54/RConn1 -- holder_1_4_solid1_1_RIGID/LConn1
  Transform53/RConn1 -- torque_nut_01_iso_1_solid1_1_RIGID/LConn1
  Transform67/RConn1 -- receptor_frsky_1_solid1_1_RIGID/LConn1
  Transform48/RConn1 -- esc_3_solid1_1_RIGID/LConn1
  Transform51/RConn1 -- plain_washer_10669_type_nl_iso_7_solid1_1_RIGID/LConn1
  Transform58/RConn1 -- plain_washer_10669_type_nl_iso_5_solid1_1_RIGID/LConn1
  Body121_1_RIGID/LConn1 -- Transform59/RConn1
  Transform68/RConn1 -- plain_washer_10669_type_nl_iso_3_solid1_1_RIGID/LConn1
  Transform69/RConn1 -- plain_washer_10669_type_nl_iso_2_solid1_1_RIGID/LConn1
  Transform64/RConn1 -- pea_gimbal4_2_1_solid1_1_RIGID/LConn1
  Transform66/RConn1 -- sec_quad_gimbal2_1_solid1_1_RIGID/LConn1
  Body106_1_RIGID/LConn1 -- Transform45/RConn1
  Transform52/RConn1 -- trem1_4_solid1_1_RIGID/LConn1
  Transform71/RConn1 -- esc_1_solid1_1_RIGID/LConn1
  Transform72/RConn1 -- veio_30_1_solid1_1_RIGID/LConn1
  Transform57/RConn1 -- plain_washer_10669_type_nl_iso_6_solid1_1_RIGID/LConn1
  Transform63/RConn1 -- servo_big40x20_1_solid1_1_RIGID/LConn1
  Body114_1_RIGID/LConn1 -- Transform55/RConn1
  Transform56/RConn1 -- torque_nut_01_iso_8_solid1_1_RIGID/LConn1
  Transform47/RConn1 -- torque_nut_01_iso_4_solid1_1_RIGID/LConn1
  Part6_2_solid1_1_RIGID/LConn1 -- Transform50/RConn1
  Transform77/RConn1 -- trem1_1_solid1_1_RIGID/LConn1
  Body15_1_RIGID/LConn1 -- Transform76/RConn1
  Transform73/RConn1 -- torque_nut_01_iso_3_solid1_1_RIGID/LConn1
  Transform78/RConn1 -- holder_1_3_solid1_1_RIGID/LConn1
  Transform75/RConn1 -- servo_arm_1_solid1_1_RIGID/LConn1
  Transform74/RConn1 -- crius_1_solid1_1_RIGID/LConn1
  Transform79/RConn1 -- torque_nut_01_iso_2_solid1_1_RIGID/LConn1
  Transform41/LConn1 -- Conn1/RConn1 -- Transform95/LConn1 -- Transform94/LConn1 -- Transform93/LConn1 -- Transform92/LConn1 -- Transform91/LConn1 -- Transform90/LConn1 -- Transform89/LConn1 -- Transform88/LConn1 -- Transform87/LConn1 -- Transform86/LConn1 -- Transform85/LConn1 -- Transform84/LConn1 -- Transform83/LConn1 -- Transform81/LConn1 -- Transform8/LConn1 -- Transform79/LConn1 -- Transform78/LConn1 -- Transform77/LConn1 -- Transform76/LConn1 -- Transform75/LConn1 -- Transform74/LConn1 -- Transform73/LConn1 -- Transform72/LConn1 -- Transform71/LConn1 -- Transform7/LConn1 -- Transform69/LConn1 -- Transform68/LConn1 -- Transform67/LConn1 -- Transform66/LConn1 -- Transform65/LConn1 -- Transform64/LConn1 -- Transform63/LConn1 -- Transform62/LConn1 -- Transform61/LConn1 -- Transform60/LConn1 -- Transform6/LConn1 -- Transform59/LConn1 -- Transform58/LConn1 -- Transform57/LConn1 -- Transform56/LConn1 -- Transform55/LConn1 -- Transform54/LConn1 -- Transform53/LConn1 -- Transform52/LConn1 -- Transform51/LConn1 -- Transform50/LConn1 -- Transform5/LConn1 -- Transform49/LConn1 -- Transform48/LConn1 -- Transform47/LConn1 -- Transform46/LConn1 -- Transform45/LConn1 -- Transform44/LConn1 -- Transform43/LConn1 -- Transform42/LConn1

== system TriTiltPro_V3/ASingle-Tilt Tricopter 3D Model/Tricopter/Frame/FrameA ==
  Body50_1_RIGID : Subsystem
  Transform{96..99} (4 alike) : sm_lib/Frames and Transforms/Rigid Transform  TranslationMethod=None  TranslationStandardOffset=0  TranslationLengthUnit=m  TranslationStandardAxis=+Z  TranslationCartesianOffset=[0 0 0]  TranslationROffset=0  TranslationROffsetUnits=m  TranslationZOffset=0  TranslationZOffsetUnits=m  TranslationThetaOffset=0  TranslationThetaOffsetUnits=deg  RotationMethod=None  RotationAngleUnits=deg  RotationStandardAxis=+Z  RotationAngle=0.0  RotationArbitraryAxis=[0 0 1]  FollAlignAxisA=+X  BaseAlignAxisA=+Y  FollAlignAxisB=+Y  BaseAlignAxisB=+Z  RotationSequenceAxes=FollowerAxes  RotationSequence=XYX  RotationSequenceAngles=[0 0 0]  RotationSequenceAnglesUnits=deg  RotationMatrix=[1 0 0; 0 1 0; 0 0 1]
  plain_washer_10669_type_nl_iso_15_solid1_1_RIGID : Subsystem
  plain_washer_10669_type_nl_iso_16_solid1_1_RIGID : Subsystem
  socket_head_cap_screw_iso_7_solid1_1_RIGID : Subsystem
  Conn1 : PMIOPort  Side=Right
  connections:
  Transform96/RConn1 -- plain_washer_10669_type_nl_iso_16_solid1_1_RIGID/LConn1
  Transform97/RConn1 -- socket_head_cap_screw_iso_7_solid1_1_RIGID/LConn1
  Body50_1_RIGID/LConn1 -- Transform98/RConn1
  Transform99/RConn1 -- plain_washer_10669_type_nl_iso_15_solid1_1_RIGID/LConn1
  Transform96/LConn1 -- Transform97/LConn1 -- Transform98/LConn1 -- Transform99/LConn1 -- Conn1/RConn1

== system TriTiltPro_V3/ASingle-Tilt Tricopter 3D Model/Tricopter/Left Rotor/ESC2 ==
  Tq : Inport
  Wmotor : Inport  Port=2
  T-W Linear Characteristic : Subsystem
  Torque-Speed DC Servomotor Linear Model : Subsystem
  Tmotor : PMIOPort  Side=Right
  Scope(Wmax) : Outport
  wires:
  Tq/1 -> Torque-Speed DC Servomotor Linear Model/1(Tmax), T-W Linear Characteristic/1(Tdemand)
  Wmotor/1 -> Torque-Speed DC Servomotor Linear Model/3(Wmotor)
  T-W Linear Characteristic/1(Wdemand) -> Scope(Wmax)/1, Torque-Speed DC Servomotor Linear Model/2(Wmax)
  connections:
  Torque-Speed DC Servomotor Linear Model/RConn1 -- Tmotor/RConn1

== system TriTiltPro_V3/ASingle-Tilt Tricopter 3D Model/Tricopter/Left Rotor/helice_gws_4_solid1_1_RIGID ==
  ReferenceFrame : sm_lib/Frames and Transforms/Reference Frame
  Solid : sm_lib/Body Elements/Solid  InertiaType=Custom  Mass=0.0068834316815648928  MassUnits=kg  CenterOfMass=[10.596314219099972 1.2795275365023604 6.1177561556766227]  CenterOfMassUnits=in  MomentsOfInertia=[0.011157453132828603 0.033180185852046074 0.022100129826974634]  MomentsOfInertiaUnits=kg*in^2  ProductsOfInertia=[-1.1628419243595612e-05 -0.015328208998132061 8.1770755294600072e-06]  ProductsOfInertiaUnits=kg*in^2  BasedOnType=Density  Density=1000  DensityUnits=kg/(m^3)  DoExposeReferenceFrame=on  SerializedFrames=<Frames/>  GraphicType=FromGeometry  MarkerShape=Sphere  MarkerSize=10  MarkerSizeUnits=m  GraphicVisPropType=SimpleVisualProperties  GraphicDiffuseColor=[1.0 0.2 0.4]  GraphicSpecularColor=[0.5 0.5 0.5 1.0]  GraphicAmbientColor=[0.15 0.15 0.15 1.0]  GraphicEmissiveColor=[0.0 0.0 0.0 1.0]  GraphicShininess=75  GraphicOpacity=1  GeometryShape=FromFile  RectangleSize=[1 1]  RectangleSizeUnits=m  BrickDimensions=[1 1 1]  BrickDimensionUnits=m  CylinderRadius=1  CylinderRadiusUnits=m  CylinderLength=1  CylinderLengthUnits=m  SphereRadius=1  SphereRadiusUnits=m  EllipsoidRadii=[1 1 1]  EllipsoidRadiiUnits=m  ExtrusionCrossSection=[1 1; -1 1; -1 -1; 1 -1]  ExtrusionCrossSectionUnits=m  ExtrusionLength=1  ExtrusionLengthUnits=m  PolygonNumSides=3  PolygonOuterRadius=1  PolygonOuterRadiusUnits=m  ExtGeomFileType=STL  ExtGeomFileName=/home/agba/Library/SImMATLAB/TRICOPTER_PROPOSALZIPPED/TRIPROSimechanicsXml_STL/helice gws-4-solid1_Default_sldprt.STL  ExtGeomFileUnits=in  RevolutionCrossSection=[1 1; 1 -1; 2 -1; 2 1]  RevolutionCrossSectionUnits=m  RevolutionExtent=Full  RevolutionAngle=180  RevolutionAngleUnits=deg
  Transform : sm_lib/Frames and Transforms/Rigid Transform  TranslationMethod=Cartesian  TranslationStandardOffset=0  TranslationLengthUnit=m  TranslationStandardAxis=+Z  TranslationCartesianOffset=[0.26915191485432344 0.037499999999999999 0.15539517080589971]  TranslationROffset=0  TranslationROffsetUnits=m  TranslationZOffset=0  TranslationZOffsetUnits=m  TranslationThetaOffset=0  TranslationThetaOffsetUnits=deg  RotationMethod=ArbitraryAxis  RotationAngleUnits=rad  RotationStandardAxis=+Z  RotationAngle=2.0943951023931953  RotationArbitraryAxis=[-0.57735026918962584 -0.57735026918962584 -0.57735026918962584]  FollAlignAxisA=+X  BaseAlignAxisA=+Y  FollAlignAxisB=+Y  BaseAlignAxisB=+Z  RotationSequenceAxes=FollowerAxes  RotationSequence=XYX  RotationSequenceAngles=[0 0 0]  RotationSequenceAnglesUnits=deg  RotationMatrix=[1 0 0; 0 1 0; 0 0 1]
  Transform1 : sm_lib/Frames and Transforms/Rigid Transform  TranslationMethod=Cartesian  TranslationStandardOffset=0  TranslationLengthUnit=m  TranslationStandardAxis=+Z  TranslationCartesianOffset=[0.26915191485432344 0.037499999999999999 0.15539517080589971]  TranslationROffset=0  TranslationROffsetUnits=m  TranslationZOffset=0  TranslationZOffsetUnits=m  TranslationThetaOffset=0  TranslationThetaOffsetUnits=deg  RotationMethod=ArbitraryAxis  RotationAngleUnits=rad  RotationStandardAxis=+Z  RotationAngle=2.0943951023931953  RotationArbitraryAxis=[0.57735026918962584 -0.57735026918962584 0.57735026918962584]  FollAlignAxisA=+X  BaseAlignAxisA=+Y  FollAlignAxisB=+Y  BaseAlignAxisB=+Z  RotationSequenceAxes=FollowerAxes  RotationSequence=XYX  RotationSequenceAngles=[0 0 0]  RotationSequenceAnglesUnits=deg  RotationMatrix=[1 0 0; 0 1 0; 0 0 1]
  F1 : PMIOPort  Side=Left
  F : PMIOPort  Port=2  Side=Right
  connections:
  Solid/RConn1 -- ReferenceFrame/RConn1 -- Transform/LConn1 -- Transform1/LConn1
  Transform/RConn1 -- F/RConn1
  Transform1/RConn1 -- F1/RConn1

== system TriTiltPro_V3/ASingle-Tilt Tricopter 3D Model/Tricopter/Left Rotor/rotor_4_solid1_1_RIGID ==
  ReferenceFrame : sm_lib/Frames and Transforms/Reference Frame
  Solid : sm_lib/Body Elements/Solid  InertiaType=Custom  Mass=0.0026802425789764052  MassUnits=kg  CenterOfMass=[10.596536889316591 0.78788999850589214 6.117913388142739]  CenterOfMassUnits=in  MomentsOfInertia=[0.00039971092252391317 0.00058906089252352132 0.00039971091362295941]  MomentsOfInertiaUnits=kg*in^2  ProductsOfInertia=[-7.0779358828117342e-12 3.7484101914791924e-11 2.4138056737191158e-11]  ProductsOfInertiaUnits=kg*in^2  BasedOnType=Density  Density=1000  DensityUnits=kg/(m^3)  DoExposeReferenceFrame=on  SerializedFrames=<Frames/>  GraphicType=FromGeometry  MarkerShape=Sphere  MarkerSize=10  MarkerSizeUnits=m  GraphicVisPropType=SimpleVisualProperties  GraphicDiffuseColor=[0.792156862745098 0.81960784313725488 0.93333333333333335]  GraphicSpecularColor=[0.5 0.5 0.5 1.0]  GraphicAmbientColor=[0.15 0.15 0.15 1.0]  GraphicEmissiveColor=[0.0 0.0 0.0 1.0]  GraphicShininess=75  GraphicOpacity=1  GeometryShape=FromFile  RectangleSize=[1 1]  RectangleSizeUnits=m  BrickDimensions=[1 1 1]  BrickDimensionUnits=m  CylinderRadius=1  CylinderRadiusUnits=m  CylinderLength=1  CylinderLengthUnits=m  SphereRadius=1  SphereRadiusUnits=m  EllipsoidRadii=[1 1 1]  EllipsoidRadiiUnits=m  ExtrusionCrossSection=[1 1; -1 1; -1 -1; 1 -1]  ExtrusionCrossSectionUnits=m  ExtrusionLength=1  ExtrusionLengthUnits=m  PolygonNumSides=3  PolygonOuterRadius=1  PolygonOuterRadiusUnits=m  ExtGeomFileType=STL  ExtGeomFileName=rotor-4-solid1_Default_sldprt.STL  ExtGeomFileUnits=in  RevolutionCrossSection=[1 1; 1 -1; 2 -1; 2 1]  RevolutionCrossSectionUnits=m  RevolutionExtent=Full  RevolutionAngle=180  RevolutionAngleUnits=deg
  Transform : sm_lib/Frames and Transforms/Rigid Transform  TranslationMethod=Cartesian  TranslationStandardOffset=0  TranslationLengthUnit=m  TranslationStandardAxis=+Z  TranslationCartesianOffset=[0.2691520371858025 0.037499999999999999 0.15539499724237449]  TranslationROffset=0  TranslationROffsetUnits=m  TranslationZOffset=0  TranslationZOffsetUnits=m  TranslationThetaOffset=0  TranslationThetaOffsetUnits=deg  RotationMethod=ArbitraryAxis  RotationAngleUnits=rad  RotationStandardAxis=+Z  RotationAngle=2.0943951023931953  RotationArbitraryAxis=[0.57735026918962584 -0.57735026918962584 0.57735026918962584]  FollAlignAxisA=+X  BaseAlignAxisA=+Y  FollAlignAxisB=+Y  BaseAlignAxisB=+Z  RotationSequenceAxes=FollowerAxes  RotationSequence=XYX  RotationSequenceAngles=[0 0 0]  RotationSequenceAnglesUnits=deg  RotationMatrix=[1 0 0; 0 1 0; 0 0 1]
  F : PMIOPort  Side=Right
  F1 : PMIOPort  Port=2  Side=Left
  connections:
  Solid/RConn1 -- ReferenceFrame/RConn1 -- Transform/LConn1 -- F1/RConn1
  Transform/RConn1 -- F/RConn1

== system TriTiltPro_V3/ASingle-Tilt Tricopter 3D Model/Tricopter/Left Rotor/spinner_4_solid1_1_RIGID ==
  ReferenceFrame : sm_lib/Frames and Transforms/Reference Frame
  Solid : sm_lib/Body Elements/Solid  InertiaType=Custom  Mass=0.00092050106035550933  MassUnits=kg  CenterOfMass=[10.596536778507584 1.6807720223174387 6.1179133081428407]  CenterOfMassUnits=in  MomentsOfInertia=[2.7129831960387464e-05 1.8078910296359469e-05 2.715753149882332e-05]  MomentsOfInertiaUnits=kg*in^2  ProductsOfInertia=[-1.932613271172059e-11 -3.8796907025777377e-08 3.2626347062310972e-11]  ProductsOfInertiaUnits=kg*in^2  BasedOnType=Density  Density=1000  DensityUnits=kg/(m^3)  DoExposeReferenceFrame=on  SerializedFrames=<Frames/>  GraphicType=FromGeometry  MarkerShape=Sphere  MarkerSize=10  MarkerSizeUnits=m  GraphicVisPropType=SimpleVisualProperties  GraphicDiffuseColor=[0.792156862745098 0.81960784313725488 0.93333333333333335]  GraphicSpecularColor=[0.5 0.5 0.5 1.0]  GraphicAmbientColor=[0.15 0.15 0.15 1.0]  GraphicEmissiveColor=[0.0 0.0 0.0 1.0]  GraphicShininess=75  GraphicOpacity=1  GeometryShape=FromFile  RectangleSize=[1 1]  RectangleSizeUnits=m  BrickDimensions=[1 1 1]  BrickDimensionUnits=m  CylinderRadius=1  CylinderRadiusUnits=m  CylinderLength=1  CylinderLengthUnits=m  SphereRadius=1  SphereRadiusUnits=m  EllipsoidRadii=[1 1 1]  EllipsoidRadiiUnits=m  ExtrusionCrossSection=[1 1; -1 1; -1 -1; 1 -1]  ExtrusionCrossSectionUnits=m  ExtrusionLength=1  ExtrusionLengthUnits=m  PolygonNumSides=3  PolygonOuterRadius=1  PolygonOuterRadiusUnits=m  ExtGeomFileType=STL  ExtGeomFileName=/home/agba/Library/SImMATLAB/TRICOPTER_PROPOSALZIPPED/TRIPROSimechanicsXml_STL/spinner-4-solid1_Default_sldprt.STL  ExtGeomFileUnits=in  RevolutionCrossSection=[1 1; 1 -1; 2 -1; 2 1]  RevolutionCrossSectionUnits=m  RevolutionExtent=Full  RevolutionAngle=180  RevolutionAngleUnits=deg
  Transform : sm_lib/Frames and Transforms/Rigid Transform  TranslationMethod=Cartesian  TranslationStandardOffset=0  TranslationLengthUnit=m  TranslationStandardAxis=+Z  TranslationCartesianOffset=[0.2691520371858025 0.037499999999999999 0.15539499724237449]  TranslationROffset=0  TranslationROffsetUnits=m  TranslationZOffset=0  TranslationZOffsetUnits=m  TranslationThetaOffset=0  TranslationThetaOffsetUnits=deg  RotationMethod=ArbitraryAxis  RotationAngleUnits=rad  RotationStandardAxis=+Z  RotationAngle=2.0943951023931953  RotationArbitraryAxis=[-0.57735026918962584 -0.57735026918962584 -0.57735026918962584]  FollAlignAxisA=+X  BaseAlignAxisA=+Y  FollAlignAxisB=+Y  BaseAlignAxisB=+Z  RotationSequenceAxes=FollowerAxes  RotationSequence=XYX  RotationSequenceAngles=[0 0 0]  RotationSequenceAnglesUnits=deg  RotationMatrix=[1 0 0; 0 1 0; 0 0 1]
  F1 : PMIOPort  Side=Left
  F : PMIOPort  Port=2  Side=Left
  connections:
  Solid/RConn1 -- ReferenceFrame/RConn1 -- Transform/LConn1 -- F1/RConn1
  Transform/RConn1 -- F/RConn1
